simulink model "dcmotor_sim_poc"  (R2018b)
settings: Solver=ode3  StartTime=0.0  StopTime=30  FixedStep=Ts  MaxStep=Ts  RelTol=1e-12  AbsTol=1e-6
values from neighbouring files (symbols this model uses):
  Ad = eye(2) + A*Ts    [makedcmotorparams.m]
  Bd = B*Ts    [makedcmotorparams.m]
  C = [1, 1]    [makedcmotorparams.m]    (also in tanks.m = [0 1])
  Cd = C    [makedcmotorparams.m]
  delta = 5e-2 * abs(spref)    [makedcmotorparams.m]
  isEvt = true    [dcmotor.m]    (also in makedcmotorparams.m)
  isg_1 = N(1,:)    [makedcmotorparams.m]
  K = place(Ad, Bd, cpoles)    [makedcmotorparams.m]
  L = place(Ad', Cd', [0.3, 0.1]).'    [makedcmotorparams.m]    (also in tanks.m = place(A', C', [-100 -2])')
  Ts = 1e-3    (= 0.001)    [makedcmotorparams.m]
  x0 = zeros(2,1)    [makedcmotorparams.m]
undefined symbols (not defined in the file or in its folder): AttackPhase
libraries: simulink x1, LinSysLib x1
settings Model: Creator=angelo  LastModifiedBy=ab1416
settings DataIOCC: ReturnWorkspaceOutputs=on  SignalLoggingName=data

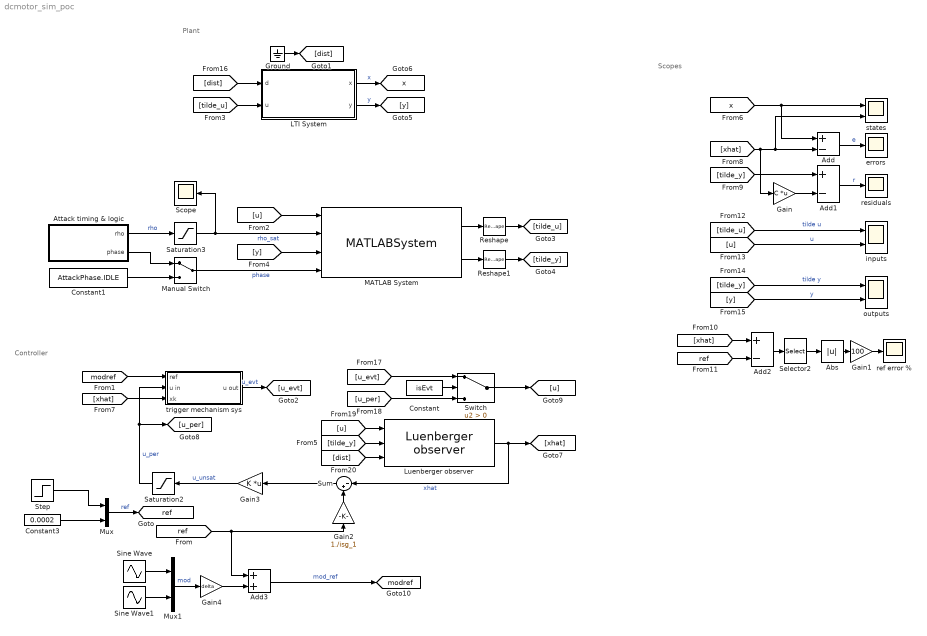
== system dcmotor_sim_poc ==
  note: Scopes
  note: Controller
  note: Plant
  Abs : Abs
  Add : Sum  Inputs=+-
  Add1 : Sum  Inputs=+-
  Add2 : Sum  Inputs=+-
  Add3 : Sum
  Attack timing & logic : Subsystem
  Constant : Constant  Value=isEvt
  Constant1 : Constant  Value=AttackPhase.IDLE
  Constant3 : Constant  Value=0.0002
  Gain : Gain  Gain=C  Multiplication=Matrix(K*u)
  Gain1 : Gain  Gain=100
  Gain2 : Gain  Gain=1./isg_1
  Gain3 : Gain  Gain=K  Multiplication=Matrix(K*u)
  Gain4 : Gain  Gain=delta
  Ground : Ground
  LTI System : Subsystem  mask{A=Ad, B=Bd, C=Cd, D=0, x0=x0}
      mask prompts: A "Matrix A:"; B "Matrix B:"; C "Matrix C:"; D "Matrix D:"; x0 "Initial condition:"
      mask help: State space model of an LTI system, with accessible state
      mask Display: disp('DT LTI System')
  Luenberger observer : LinSysLib/Discrete time/Luenberger observer  A=Ad  B=Bd  C=Cd  D=0  hatx0=x0  L=L
  MATLAB System : MATLABSystem  System=ReplayAttacker  bufferSize=1024*1024  SimulateUsing=Code generation
      mask Type: ReplayAttacker
      mask Display:
      | disp('ReplayAttacker');
      | port_label('input',1,'u');
      | port_label('input',2,'rho');
      | port_label('input',3,'y');
      | port_label('input',4,'phase');
      | port_label('output',1,'tildeu');
      | port_label('output',2,'tildey');
  Manual Switch : ManualSwitch
  Mux : Mux  Inputs=2
  Mux1 : Mux  Inputs=2
  Reshape : Reshape  OutputDimensionality=Customize  OutputDimensions=1
  Reshape1 : Reshape  OutputDimensionality=Customize  OutputDimensions=1
  Saturation2 : Saturate  UpperLimit=20  LowerLimit=-20
  Saturation3 : Saturate  UpperLimit=20  LowerLimit=-20
  Scope : Scope
  Selector2 : Selector  InputPortWidth=2  IndexOptions=Index vector (dialog)  Indices=1  OutputSizes=1
  Sine Wave : Sin  SampleTime=Ts
  Sine Wave1 : Sin  Phase=pi/2  SampleTime=Ts
  Step : Step  Time=0  SampleTime=Ts
  Sum : Sum  Inputs=|-+
  Switch : Switch  Criteria=u2 > Threshold
  errors : Scope
  inputs : Scope  NumInputPorts=2
  outputs : Scope  NumInputPorts=2
  ref error % : Scope
  residuals : Scope
  states : Scope  NumInputPorts=2
  trigger mechanism sys : Subsystem
  tag scope: modref=global, ref=global, x=global
  wires:
  [xhat] -> Gain/1, Add/2, states/2
  [x] -> states/1, Add/1
  Add/1 -> errors/1  "e"
  Sum/1 -> Gain3/1
  Mux/1 -> [ref]  "ref"
  [modref] -> trigger mechanism sys/1(ref)
  LTI System/2(y) -> [y]  "y"
  LTI System/1(x) -> [x]  "x"
  [tilde_y] -> Luenberger observer/2
  [xhat] -> trigger mechanism sys/3(xk)
  [tilde_y] -> Add1/1
  Gain/1 -> Add1/2
  Add1/1 -> residuals/1  "r"
  Selector2/1 -> Abs/1
  Gain1/1 -> ref error %/1
  Abs/1 -> Gain1/1
  [u] -> MATLAB System/1
  MATLAB System/1 -> Reshape/1
  MATLAB System/2 -> Reshape1/1
  [y] -> MATLAB System/3
  [u] -> inputs/2  "u"
  [tilde_u] -> inputs/1  "tilde u"
  [tilde_y] -> outputs/1  "tilde y"
  [y] -> outputs/2  "y"
  Manual Switch/1 -> MATLAB System/4  "phase"
  Constant1/1 -> Manual Switch/2
  trigger mechanism sys/1(u out) -> [u_evt]  "u_evt"
  Gain3/1 -> Saturation2/1  "u_unsat"
  [u] -> Luenberger observer/1
  Constant3/1 -> Mux/2
  [xhat] -> Add2/1
  [ref] -> Add2/2
  Add2/1 -> Selector2/1
  Step/1 -> Mux/1
  [tilde_u] -> LTI System/2(u)
  Saturation2/1 -> trigger mechanism sys/2(u in), [u_per]  "u_per"
  Attack timing & logic/1(rho) -> Saturation3/1  "rho"
  Attack timing & logic/2(phase) -> Manual Switch/1
  Saturation3/1 -> MATLAB System/2, Scope/1  "rho_sat"
  Ground/1 -> [dist]
  [dist] -> LTI System/1(d)
  [dist] -> Luenberger observer/3
  Luenberger observer/1 -> Sum/1, [xhat]  "xhat"
  [u_per] -> Switch/3
  [u_evt] -> Switch/1
  Constant/1 -> Switch/2
  Switch/1 -> [u]
  Gain2/1 -> Sum/2
  Reshape/1 -> [tilde_u]
  Reshape1/1 -> [tilde_y]
  [ref] -> Gain2/1, Add3/1
  Add3/1 -> [modref]  "mod_ref"
  Gain4/1 -> Add3/2
  Mux1/1 -> Gain4/1  "mod"
  Sine Wave/1 -> Mux1/1
  Sine Wave1/1 -> Mux1/2

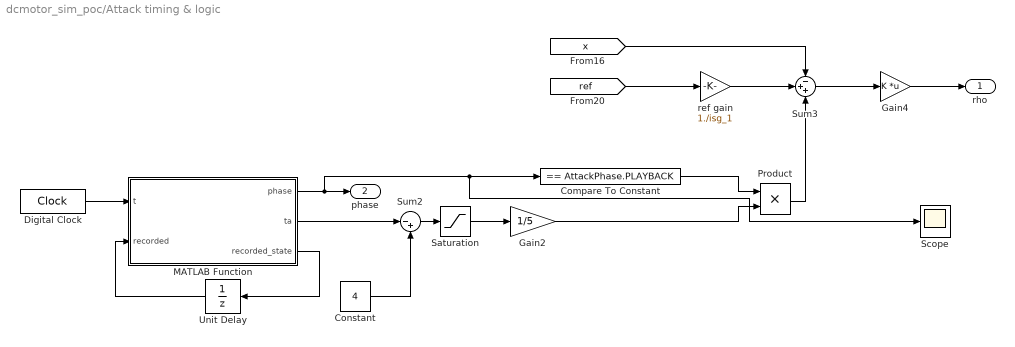
== system dcmotor_sim_poc/Attack timing & logic ==
  Compare To Constant : simulink/Logic and Bit Operations/Compare To Constant  relop===  const=AttackPhase.PLAYBACK  OutDataTypeStr=boolean
  Constant : Constant  Value=4
  Digital Clock : DigitalClock  SampleTime=Ts
  Gain2 : Gain  Gain=1/5
  Gain4 : Gain  Gain=K  Multiplication=Matrix(K*u)
  MATLAB Function : MATLAB Function  TreatAsAtomicUnit=on
  Product : Product
  Saturation : Saturate  UpperLimit=inf  LowerLimit=0
  Scope : Scope
  Sum2 : Sum  Inputs=|-+
  Sum3 : Sum  Inputs=-++
  Unit Delay : UnitDelay  SampleTime=Ts
  ref gain : Gain  Gain=1./isg_1
  rho : Outport  VectorParamsAs1DForOutWhenUnconnected=on
  phase : Outport  Port=2  VectorParamsAs1DForOutWhenUnconnected=on
  wires:
  Sum3/1 -> Gain4/1
  Compare To Constant/1 -> Product/1
  Digital Clock/1 -> MATLAB Function/1(t)
  MATLAB Function/1(phase) -> Scope/1, Compare To Constant/1, phase/1
  Gain2/1 -> Product/2
  MATLAB Function/2(ta) -> Sum2/1
  Gain4/1 -> rho/1
  [ref] -> ref gain/1
  ref gain/1 -> Sum3/2
  Unit Delay/1 -> MATLAB Function/2(recorded)
  Constant/1 -> Sum2/2
  MATLAB Function/3(recorded_state) -> Unit Delay/1
  Product/1 -> Sum3/3
  Saturation/1 -> Gain2/1
  [x] -> Sum3/1
  Sum2/1 -> Saturation/1

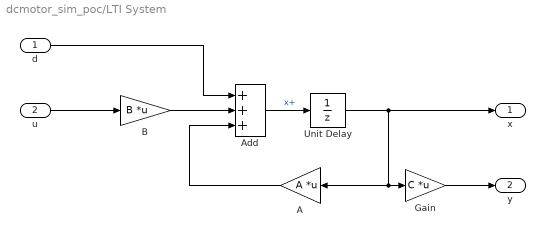
== system dcmotor_sim_poc/LTI System ==
  d : Inport
  u : Inport  Port=2  PortDimensions=size(B,2)
  A : Gain  Gain=A  Multiplication=Matrix(K*u)
  Add : Sum  Inputs=+++
  B : Gain  Gain=B  Multiplication=Matrix(K*u)
  Gain : Gain  Gain=C  Multiplication=Matrix(K*u)
  Unit Delay : UnitDelay  InitialCondition=x0  SampleTime=-1
  x : Outport  PortDimensions=size(A,1)
  y : Outport  Port=2  PortDimensions=size(C,1)
  wires:
  d/1 -> Add/1
  Gain/1 -> y/1
  A/1 -> Add/3
  Add/1 -> Unit Delay/1  "x+"
  Unit Delay/1 -> Gain/1, A/1, x/1
  B/1 -> Add/2
  u/1 -> B/1

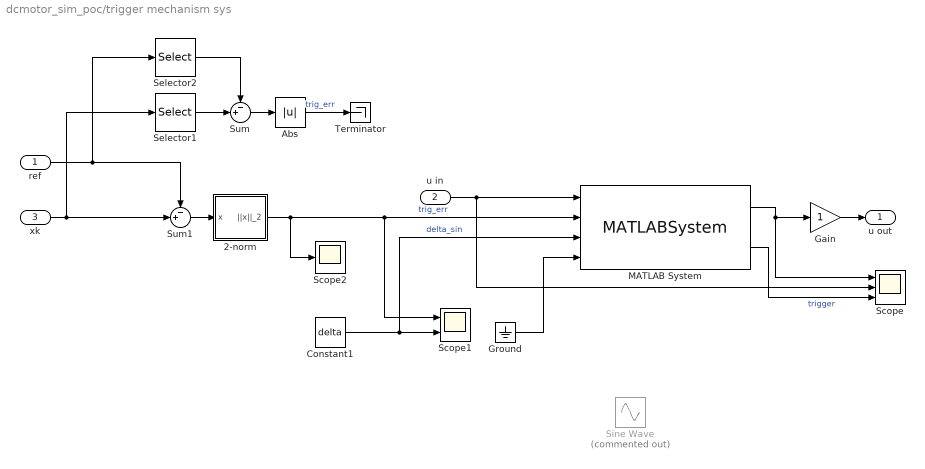
== system dcmotor_sim_poc/trigger mechanism sys ==
  ref : Inport
  u in : Inport  Port=2  PortDimensions=1
  xk : Inport  Port=3
  2-norm : Subsystem
  Abs : Abs
  Constant1 : Constant  Value=delta
  Gain : Gain
  Ground : Ground
  MATLAB System : MATLABSystem  System=TriggerSystem  SimulateUsing=Code generation
      mask Type: TriggerSystem
      mask Display:
      | disp('TriggerSystem');
      | port_label('input',1,'u');
      | port_label('input',2,'err');
      | port_label('input',3,'delta');
      | port_label('input',4,'aux');
      | port_label('output',1,'uTrig');
      | port_label('output',2,'trig');
  Scope : Scope  NumInputPorts=3
  Scope1 : Scope  NumInputPorts=2
  Scope2 : Scope
  Selector1 : Selector  InputPortWidth=2  IndexOptions=Index vector (dialog)  Indices=1  OutputSizes=1
  Selector2 : Selector  InputPortWidth=2  IndexOptions=Index vector (dialog)  Indices=1  OutputSizes=1
  Sine Wave : Sin  Commented=on  Amplitude=delta  Bias=delta  Frequency=10  SampleTime=Ts
  Sum : Sum  Inputs=-+|
  Sum1 : Sum  Inputs=-+|
  Terminator : Terminator
  u out : Outport  VectorParamsAs1DForOutWhenUnconnected=on
  wires:
  u in/1 -> MATLAB System/1, Scope/2
  2-norm/1(||x||_2) -> Scope1/1, MATLAB System/2, Scope2/1  "trig_err"
  xk/1 -> Selector1/1, Sum1/2
  Sum/1 -> Abs/1
  Selector1/1 -> Sum/2
  Selector2/1 -> Sum/1
  MATLAB System/1 -> Scope/1, Gain/1
  MATLAB System/2 -> Scope/3  "trigger"
  ref/1 -> Selector2/1, Sum1/1
  Constant1/1 -> Scope1/2, MATLAB System/3  "delta_sin"
  Gain/1 -> u out/1
  Sum1/1 -> 2-norm/1(x)
  Ground/1 -> MATLAB System/4
  Abs/1 -> Terminator/1  "trig_err"

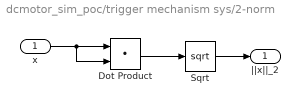
== system dcmotor_sim_poc/trigger mechanism sys/2-norm ==
  x : Inport
  Dot Product : DotProduct  InputSameDT=on  OutDataTypeStr=Inherit: Inherit via internal rule
  Sqrt : Sqrt  SaturateOnIntegerOverflow=on
  ||x||_2 : Outport
  wires:
  x/1 -> Dot Product/2, Dot Product/1
  Dot Product/1 -> Sqrt/1
  Sqrt/1 -> ||x||_2/1

== matlab function dcmotor_sim_poc/Attack timing & logic/MATLAB Function ==
  data: t input; phase output Enum: AttackPhase size=1; ta output; recorded input; recorded_state output
function [phase, ta, recorded_state] = attackSchedule(t, recorded)

kr = 5;
Tr = 10;
Ta = 8;
ka = 20;

h = mod(t,40);

if h > kr && h <= kr + Tr && recorded == 0
    phase = AttackPhase.RECORD;
    ta = 10;
    recorded_state = recorded;
elseif h > ka && h <= ka + Ta
    phase = AttackPhase.PLAYBACK;
    ta = h - ka;
    recorded_state = 1;
else
    phase = AttackPhase.IDLE;
    ta = 10;
    recorded_state = recorded;
end


end
